simulink model "Simulations_chapter5_method2"  (R2023a)
settings: Solver=ode23s  StartTime=0.0  StopTime=20  RelTol=1e-3  EnableMultiTasking=on
values from neighbouring files (symbols this model uses):
  Akmax = EstMax.a    [Chapter5_method2.m]
  Akmin = Estmin.a    [Chapter5_method2.m]
  Bkmax = EstMax.b    [Chapter5_method2.m]
  Bkmin = Estmin.b    [Chapter5_method2.m]
  c0 = 68.83    [Chapter5_method2.m]
  c1 = 21    [Chapter5_method2.m]
  Ckmax = EstMax.c    [Chapter5_method2.m]
  Ckmin = Estmin.c    [Chapter5_method2.m]
  Dkmax = EstMax.d    [Chapter5_method2.m]
  Dkmin = Estmin.d    [Chapter5_method2.m]
  fc = 28.07    [Chapter5_method2.m]
  Fer0 = 1    [Init_simulations_chapter5_method2.m]
  k0 = 170.4    [Chapter5_method2.m]
  k1 = 218.16    [Chapter5_method2.m]
  ks = 1396    [Chapter5_method2.m]
  kt = 12270    [Chapter5_method2.m]
  ms = 2.27    [Chapter5_method2.m]
  mus = 0.25    [Chapter5_method2.m]
  rhomax = 1    [Chapter5_method2.m]
  rhomin = -1    [Chapter5_method2.m]
  scenario = input('Which scenario would you like to run: 1, 2 or 3? Answer = ')    [Init_simulations_chapter5_method2.m]
  tau = 43e-3    (= 0.043)    [Chapter5_method2.m]
  Ts = 0.005    [Init_simulations_chapter5_method2.m]
  umax = 0.35    [Init_simulations_chapter5_method2.m]
  umin = 0.1    [Init_simulations_chapter5_method2.m]
  zs0 = 0.001    [Init_simulations_chapter5_method2.m]
  zsdt0 = 0.001    [Init_simulations_chapter5_method2.m]
  zus0 = 0.001    [Init_simulations_chapter5_method2.m]
  zusdt0 = 0.001    [Init_simulations_chapter5_method2.m]
libraries: simulink x4
settings Model: Creator=aestr  LastModifiedBy=senameo
settings SolverCC: AlgebraicLoopSolver=TrustRegion
settings DataIOCC: LimitDataPoints=on  SaveFormat=Array  ReturnWorkspaceOutputs=off
settings OptimizationCC: LifeSpan=inf
settings DebuggingCC: UnconnectedInputMsg=warning  UnconnectedOutputMsg=warning  UnconnectedLineMsg=warning  SFUnexpectedBacktrackingDiag=warning  SFNoUnconditionalDefaultTransitionDiag=warning  SFExecutionAtInitializationDiag=none  ArithmeticOperatorsInVariantConditions=warning
settings HardwareCC: ProdBitPerPointer=32  ProdBitPerSizeT=32  ProdBitPerPtrDiffT=32  ProdLargestAtomicFloat=None  ProdIntDivRoundTo=Undefined  ProdEndianess=Unspecified  ProdWordSize=32  ProdHWDeviceType=32-bit Generic
settings ModelReferenceCC: EnableRefExpFcnMdlSchedulingChecks=on  PropagateSignalLabelsOutOfModel=off
settings SFSimCC: SimUseLocalCustomCode=off  CustomCodeUndefinedFunction=UseInterfaceOnly
settings RTWCC: RTWUseLocalCustomCode=off  DLArmComputeVersion=19.05
settings CodeAppCC: StateflowObjectComments=on
settings GRTTargetCC: TargetLangStandard=C89/C90 (ANSI)
settings ConfigComp: CovMetricSettings=dw  CovSaveCumulativeToWorkspaceVar=on  CovSaveSingleToWorkspaceVar=on  CovExternalEMLEnable=off

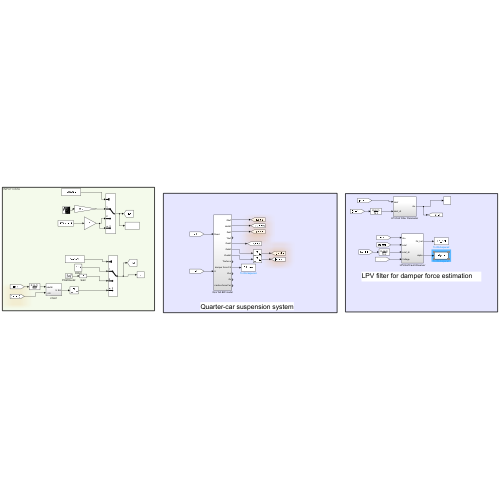
[thumbnail: Simulink's stored preview of the top-level diagram]
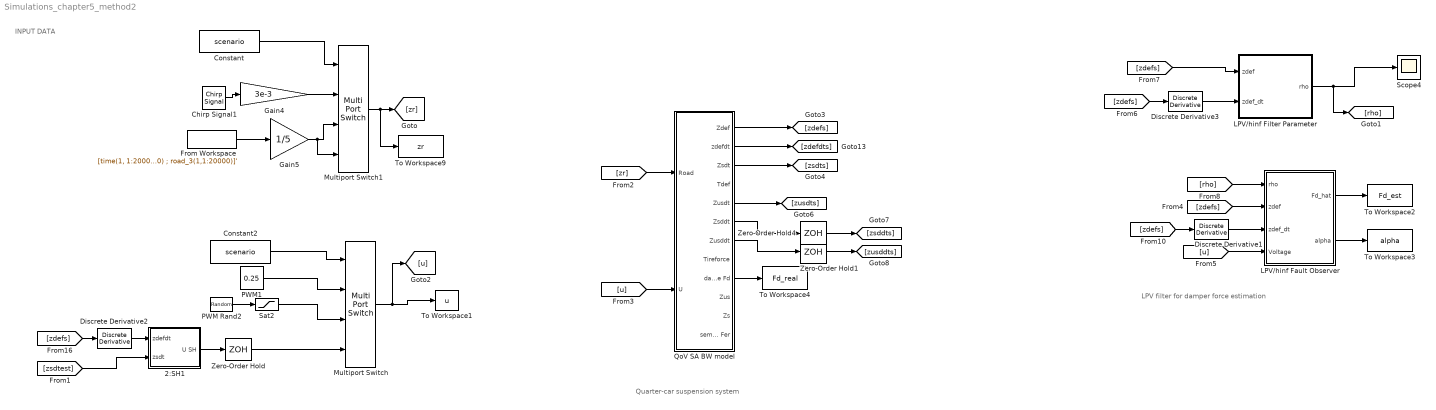
== system Simulations_chapter5_method2 ==
  note: INPUT DATA
  note: Quarter-car suspension system
  note: LPV filter for damper force estimation
  2:SH1 : Subsystem  AncestorBlock=controladores/Hybrid Controller/Sky Hook
  Chirp Signal1 : simulink/Sources/Chirp Signal  f1=0  T=20  f2=10
  Constant : Constant  Value=scenario
  Constant2 : Constant  Value=scenario
  Discrete Derivative1 : simulink/Discrete/Discrete Derivative  gainval=1.0  ICPrevScaledInput=0.0  OutMin=[]  OutMax=[]  OutDataType=fixdt(1, 16)  OutScaling=2^-10  DoSatur=off
  Discrete Derivative2 : simulink/Discrete/Discrete Derivative  gainval=1.0  ICPrevScaledInput=0.0  OutMin=[]  OutMax=[]  OutDataType=fixdt(1, 16)  OutScaling=2^-10  DoSatur=off
  Discrete Derivative3 : simulink/Discrete/Discrete Derivative  gainval=1.0  ICPrevScaledInput=0.0  OutMin=[]  OutMax=[]  OutDataType=fixdt(1, 16)  OutScaling=2^-10  DoSatur=off
  From Workspace : FromWorkspace  VariableName=[time(1, 1:20000) ; road_3(1,1:20000)]'
  Gain4 : Gain  Gain=3e-3
  Gain5 : Gain  Gain=1/5
  LPV/hinf Fault Observer : Subsystem
  LPV/hinf Filter Parameter : Subsystem
  Multiport Switch : MultiPortSwitch  SaturateOnIntegerOverflow=off  InputSameDT=off
  Multiport Switch1 : MultiPortSwitch  SaturateOnIntegerOverflow=off  InputSameDT=off
  PWM Rand2 : UniformRandomNumber  Minimum=0.05  Maximum=0.4  Seed=5  SampleTime=2
  PWM1 : Constant  Value=0.25
  QoV SA BW model : Subsystem
  Sat2 : Saturate  UpperLimit=0.35  LowerLimit=0.1
  Scope4 : Scope
  To Workspace1 : ToWorkspace  VariableName=u  SaveFormat=Structure With Time  SampleTime=-1
  To Workspace2 : ToWorkspace  VariableName=Fd_est  SaveFormat=Structure With Time  SampleTime=-1
  To Workspace3 : ToWorkspace  VariableName=alpha  SaveFormat=Structure With Time  SampleTime=-1
  To Workspace4 : ToWorkspace  VariableName=Fd_real  SaveFormat=Structure With Time  SampleTime=-1
  To Workspace9 : ToWorkspace  VariableName=zr  SaveFormat=Structure With Time  SampleTime=-1
  Zero-Order Hold : ZeroOrderHold  SampleTime=Ts
  Zero-Order Hold1 : ZeroOrderHold  SampleTime=Ts
  Zero-Order Hold4 : ZeroOrderHold  SampleTime=Ts
  wires:
  QoV SA BW model/3(Zsdt) -> [zsdts]
  QoV SA BW model/5(Zusdt) -> [zusdts]
  QoV SA BW model/7(Zusddt) -> Zero-Order Hold1/1
  Zero-Order Hold4/1 -> [zsddts]
  Zero-Order Hold1/1 -> [zusddts]
  QoV SA BW model/9(damper force Fd) -> To Workspace4/1
  QoV SA BW model/2(zdefdt) -> [zdefdts]
  QoV SA BW model/1(Zdef) -> [zdefs]
  QoV SA BW model/6(Zsddt) -> Zero-Order Hold4/1
  Multiport Switch1/1 -> To Workspace9/1, [zr]
  Chirp Signal1/1 -> Gain4/1
  [zr] -> QoV SA BW model/1(Road)
  [u] -> QoV SA BW model/2(U)
  [zdefs] -> Discrete Derivative2/1
  Discrete Derivative2/1 -> 2:SH1/1(zdefdt)
  [zsdtest] -> 2:SH1/2(zsdt)
  Constant2/1 -> Multiport Switch/1
  2:SH1/1(U SH) -> Zero-Order Hold/1
  Sat2/1 -> Multiport Switch/3
  PWM1/1 -> Multiport Switch/2
  Multiport Switch/1 -> To Workspace1/1, [u]
  Zero-Order Hold/1 -> Multiport Switch/4
  PWM Rand2/1 -> Sat2/1
  Constant/1 -> Multiport Switch1/1
  Gain4/1 -> Multiport Switch1/2
  From Workspace/1 -> Gain5/1
  Gain5/1 -> Multiport Switch1/4, Multiport Switch1/3
  Discrete Derivative3/1 -> LPV/hinf Filter Parameter/2(zdef_dt)
  [zdefs] -> Discrete Derivative3/1
  LPV/hinf Filter Parameter/1(rho) -> [rho], Scope4/1
  [zdefs] -> LPV/hinf Filter Parameter/1(zdef)
  Discrete Derivative1/1 -> LPV/hinf Fault Observer/3(zdef_dt)
  [zdefs] -> LPV/hinf Fault Observer/2(zdef)
  [zdefs] -> Discrete Derivative1/1
  [u] -> LPV/hinf Fault Observer/4(Voltage)
  [rho] -> LPV/hinf Fault Observer/1(rho)
  LPV/hinf Fault Observer/1(Fd_hat) -> To Workspace2/1
  LPV/hinf Fault Observer/2(alpha) -> To Workspace3/1

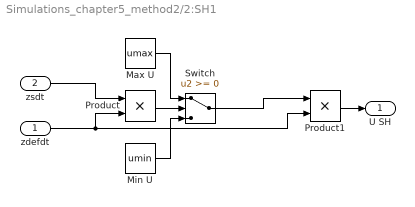
== system Simulations_chapter5_method2/2:SH1 ==
  zdefdt : Inport
  zsdt : Inport  Port=2
  Max U : Constant  Value=umax
  Min U : Constant  Value=umin
  Product : Product  RndMeth=Zero
  Product1 : Product  RndMeth=Zero
  Switch : Switch  SaturateOnIntegerOverflow=off  InputSameDT=off
  U SH : Outport  VectorParamsAs1DForOutWhenUnconnected=off
  wires:
  zsdt/1 -> Product/1
  zdefdt/1 -> Product1/2, Product/2
  Max U/1 -> Switch/1
  Min U/1 -> Switch/3
  Product/1 -> Switch/2
  Switch/1 -> Product1/1
  Product1/1 -> U SH/1

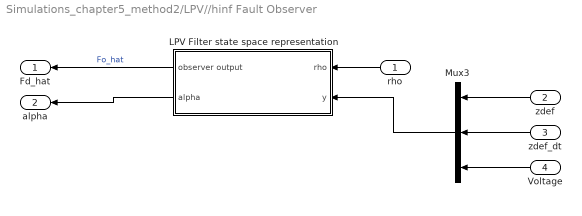
== system Simulations_chapter5_method2/LPV//hinf Fault Observer ==
  rho : Inport
  zdef : Inport  Port=2
  zdef_dt : Inport  Port=3
  Voltage : Inport  Port=4
  LPV Filter state space representation : Subsystem
  Mux3 : Mux  Inputs=3
  Fd_hat : Outport
  alpha : Outport  Port=2
  wires:
  Mux3/1 -> LPV Filter state space representation/2(y)
  LPV Filter state space representation/1(observer output) -> Fd_hat/1  "Fo_hat"
  Voltage/1 -> Mux3/3
  zdef/1 -> Mux3/1
  zdef_dt/1 -> Mux3/2
  LPV Filter state space representation/2(alpha) -> alpha/1
  rho/1 -> LPV Filter state space representation/1(rho)

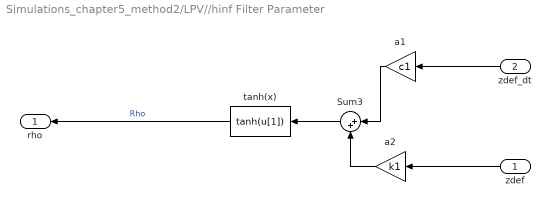
== system Simulations_chapter5_method2/LPV//hinf Filter Parameter ==
  zdef : Inport
  zdef_dt : Inport  Port=2
  Sum3 : Sum  Inputs=|++
  a1 : Gain  Gain=c1
  a2 : Gain  Gain=k1
  tanh(x) : Fcn  Expr=tanh(u[1])
  rho : Outport
  wires:
  Sum3/1 -> tanh(x)/1
  a2/1 -> Sum3/2
  a1/1 -> Sum3/1
  tanh(x)/1 -> rho/1  "Rho"
  zdef/1 -> a2/1
  zdef_dt/1 -> a1/1

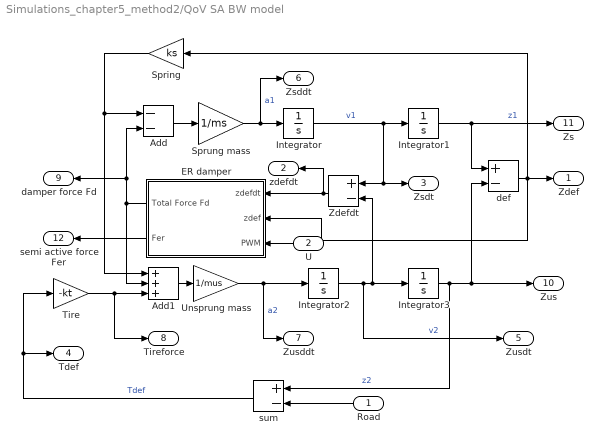
== system Simulations_chapter5_method2/QoV SA BW model ==
  Road : Inport
  U : Inport  Port=2
  Add : Sum  Inputs=--
  Add1 : Sum  Inputs=+++
  ER damper : Subsystem
  Integrator : Integrator  InitialCondition=zsdt0
  Integrator1 : Integrator  InitialCondition=zs0
  Integrator2 : Integrator  InitialCondition=zusdt0
  Integrator3 : Integrator  InitialCondition=zus0
  Spring : Gain  Gain=ks
  Sprung mass : Gain  Gain=1/ms
  Tire : Gain  Gain=-kt
  Unsprung mass : Gain  Gain=1/mus
  Zdefdt : Sum  Inputs=+-
  def : Sum  Inputs=+-
  sum : Sum  Inputs=+-
  Zdef : Outport
  zdefdt : Outport  Port=2
  Zsdt : Outport  Port=3
  Tdef : Outport  Port=4
  Zusdt : Outport  Port=5
  Zsddt : Outport  Port=6
  Zusddt : Outport  Port=7
  Tireforce : Outport  Port=8
  damper force Fd : Outport  Port=9
  Zus : Outport  Port=10
  Zs : Outport  Port=11
  semi active force Fer : Outport  Port=12
  wires:
  Integrator/1 -> Zsdt/1, Zdefdt/1, Integrator1/1  "v1"
  Integrator2/1 -> Zusdt/1, Zdefdt/2, Integrator3/1  "v2"
  Sprung mass/1 -> Zsddt/1, Integrator/1  "a1"
  Unsprung mass/1 -> Zusddt/1, Integrator2/1  "a2"
  Add/1 -> Sprung mass/1
  Add1/1 -> Unsprung mass/1
  Integrator1/1 -> def/1, Zs/1  "z1"
  Integrator3/1 -> sum/1, def/2, Zus/1  "z2"
  def/1 -> ER damper/2(zdef), Zdef/1, Spring/1
  Spring/1 -> Add/1, Add1/1
  Tire/1 -> Tireforce/1, Add1/3
  Road/1 -> sum/2
  sum/1 -> Tdef/1, Tire/1  "Tdef"
  ER damper/1(Total Force Fd) -> Add1/2, Add/2, damper force Fd/1
  U/1 -> ER damper/3(PWM)
  Zdefdt/1 -> ER damper/1(zdefdt), zdefdt/1
  ER damper/2(Fer) -> semi active force Fer/1

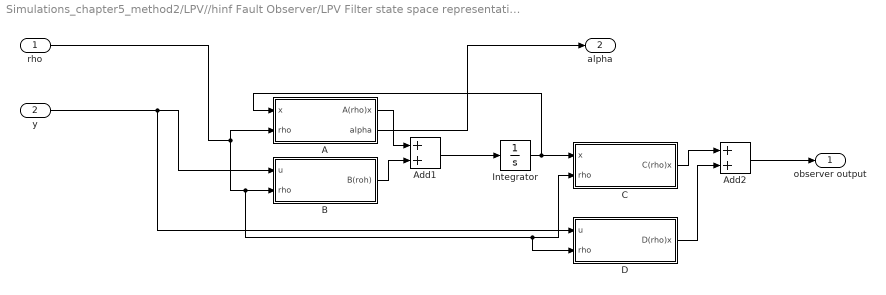
== system Simulations_chapter5_method2/LPV//hinf Fault Observer/LPV Filter state space representation ==
  rho : Inport
  y : Inport  Port=2
  A : Subsystem
  Add1 : Sum
  Add2 : Sum
  B : Subsystem
  C : Subsystem
  D : Subsystem
  Integrator : Integrator
  observer output : Outport  VectorParamsAs1DForOutWhenUnconnected=off
  alpha : Outport  Port=2  VectorParamsAs1DForOutWhenUnconnected=off
  wires:
  A/2(alpha) -> alpha/1
  C/1(C(rho)x) -> Add2/1
  D/1(D(rho)x) -> Add2/2
  Integrator/1 -> C/1(x), A/1(x)
  Add1/1 -> Integrator/1
  B/1(B(roh)) -> Add1/2
  A/1(A(rho)x) -> Add1/1
  rho/1 -> A/2(rho), B/2(rho), C/2(rho), D/2(rho)
  Add2/1 -> observer output/1
  y/1 -> B/1(u), D/1(u)

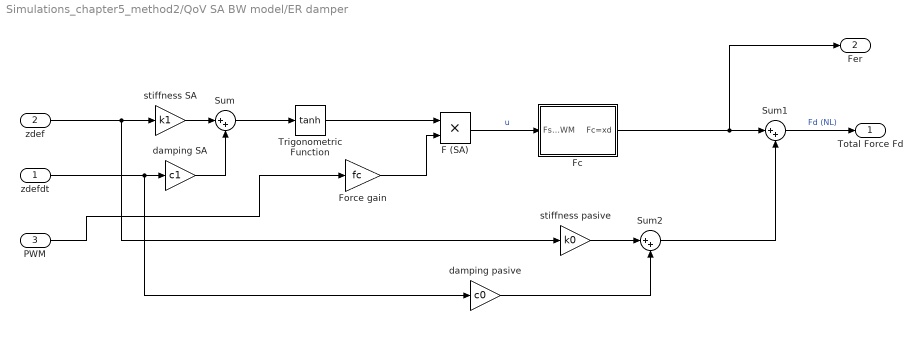
== system Simulations_chapter5_method2/QoV SA BW model/ER damper ==
  zdefdt : Inport
  zdef : Inport  Port=2
  PWM : Inport  Port=3
  "F (SA) " : Product  RndMeth=Zero
  Fc : Subsystem
  Force gain : Gain  Gain=fc
  Sum : Sum  Inputs=|++
  Sum1 : Sum  Inputs=|++
  Sum2 : Sum  Inputs=|++
  Trigonometric Function : Trigonometry  Operator=tanh
  damping SA : Gain  Gain=c1
  damping pasive : Gain  Gain=c0
  stiffness SA : Gain  Gain=k1
  stiffness pasive : Gain  Gain=k0
  Total Force Fd : Outport
  Fer : Outport  Port=2
  wires:
  zdefdt/1 -> damping pasive/1, damping SA/1
  stiffness SA/1 -> Sum/1
  damping SA/1 -> Sum/2
  Sum/1 -> Trigonometric Function/1
  Trigonometric Function/1 -> "F (SA) "/1
  PWM/1 -> Force gain/1
  Force gain/1 -> "F (SA) "/2
  stiffness pasive/1 -> Sum2/1
  damping pasive/1 -> Sum2/2
  "F (SA) "/1 -> Fc/1(Fsa*PWM)  "u"
  Fc/1(Fc=xd) -> Fer/1, Sum1/1
  Sum2/1 -> Sum1/2
  Sum1/1 -> Total Force Fd/1  "Fd (NL)"
  zdef/1 -> stiffness pasive/1, stiffness SA/1

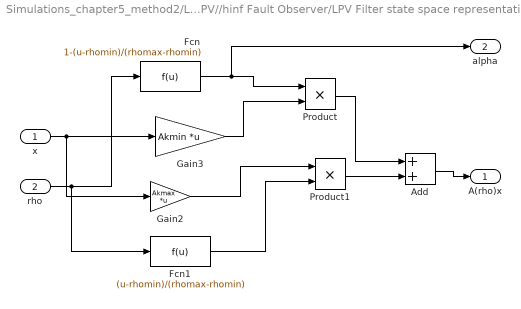
== system Simulations_chapter5_method2/LPV//hinf Fault Observer/LPV Filter state space representation/A ==
  x : Inport
  rho : Inport  Port=2
  Add : Sum
  Fcn : Fcn  Expr=1-(u-rhomin)/(rhomax-rhomin)
  Fcn1 : Fcn  Expr=(u-rhomin)/(rhomax-rhomin)
  Gain2 : Gain  Gain=Akmax  Multiplication=Matrix(K*u)
  Gain3 : Gain  Gain=Akmin  Multiplication=Matrix(K*u)
  Product : Product
  Product1 : Product
  A(rho)x : Outport  VectorParamsAs1DForOutWhenUnconnected=off
  alpha : Outport  Port=2  VectorParamsAs1DForOutWhenUnconnected=off
  wires:
  x/1 -> Gain3/1, Gain2/1
  rho/1 -> Fcn/1, Fcn1/1
  Product/1 -> Add/1
  Product1/1 -> Add/2
  Add/1 -> A(rho)x/1
  Fcn/1 -> Product/1, alpha/1
  Fcn1/1 -> Product1/2
  Gain3/1 -> Product/2
  Gain2/1 -> Product1/1

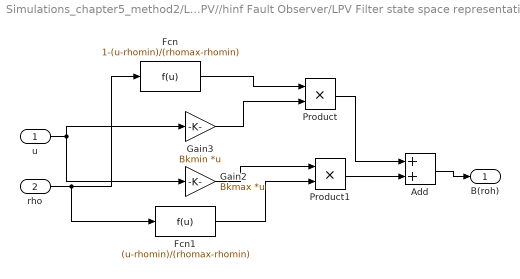
== system Simulations_chapter5_method2/LPV//hinf Fault Observer/LPV Filter state space representation/B ==
  u : Inport
  rho : Inport  Port=2
  Add : Sum
  Fcn : Fcn  Expr=1-(u-rhomin)/(rhomax-rhomin)
  Fcn1 : Fcn  Expr=(u-rhomin)/(rhomax-rhomin)
  Gain2 : Gain  Gain=Bkmax  Multiplication=Matrix(K*u)
  Gain3 : Gain  Gain=Bkmin  Multiplication=Matrix(K*u)
  Product : Product
  Product1 : Product
  B(roh) : Outport  VectorParamsAs1DForOutWhenUnconnected=off
  wires:
  u/1 -> Gain3/1, Gain2/1
  rho/1 -> Fcn/1, Fcn1/1
  Product/1 -> Add/1
  Product1/1 -> Add/2
  Add/1 -> B(roh)/1
  Fcn/1 -> Product/1
  Fcn1/1 -> Product1/2
  Gain3/1 -> Product/2
  Gain2/1 -> Product1/1

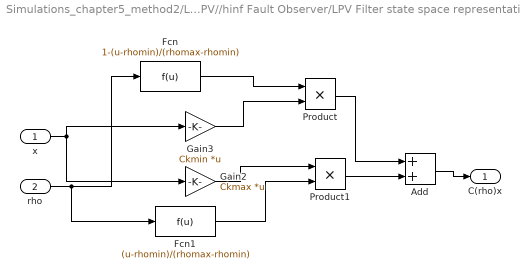
== system Simulations_chapter5_method2/LPV//hinf Fault Observer/LPV Filter state space representation/C ==
  x : Inport
  rho : Inport  Port=2
  Add : Sum
  Fcn : Fcn  Expr=1-(u-rhomin)/(rhomax-rhomin)
  Fcn1 : Fcn  Expr=(u-rhomin)/(rhomax-rhomin)
  Gain2 : Gain  Gain=Ckmax  Multiplication=Matrix(K*u)
  Gain3 : Gain  Gain=Ckmin  Multiplication=Matrix(K*u)
  Product : Product
  Product1 : Product
  C(rho)x : Outport  VectorParamsAs1DForOutWhenUnconnected=off
  wires:
  x/1 -> Gain3/1, Gain2/1
  rho/1 -> Fcn/1, Fcn1/1
  Product/1 -> Add/1
  Product1/1 -> Add/2
  Add/1 -> C(rho)x/1
  Fcn/1 -> Product/1
  Fcn1/1 -> Product1/2
  Gain3/1 -> Product/2
  Gain2/1 -> Product1/1

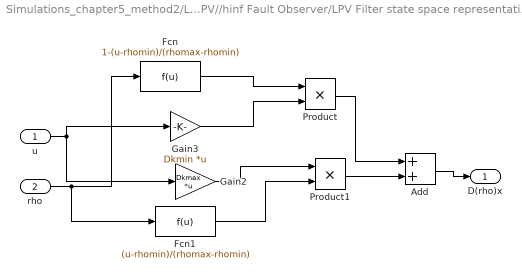
== system Simulations_chapter5_method2/LPV//hinf Fault Observer/LPV Filter state space representation/D ==
  u : Inport
  rho : Inport  Port=2
  Add : Sum
  Fcn : Fcn  Expr=1-(u-rhomin)/(rhomax-rhomin)
  Fcn1 : Fcn  Expr=(u-rhomin)/(rhomax-rhomin)
  Gain2 : Gain  Gain=Dkmax  Multiplication=Matrix(K*u)
  Gain3 : Gain  Gain=Dkmin  Multiplication=Matrix(K*u)
  Product : Product
  Product1 : Product
  D(rho)x : Outport  VectorParamsAs1DForOutWhenUnconnected=off
  wires:
  u/1 -> Gain3/1, Gain2/1
  rho/1 -> Fcn/1, Fcn1/1
  Product/1 -> Add/1
  Product1/1 -> Add/2
  Add/1 -> D(rho)x/1
  Fcn/1 -> Product/1
  Fcn1/1 -> Product1/2
  Gain3/1 -> Product/2
  Gain2/1 -> Product1/1

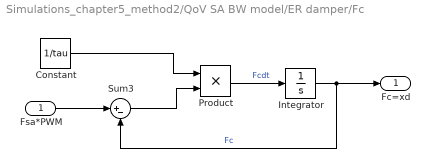
== system Simulations_chapter5_method2/QoV SA BW model/ER damper/Fc ==
  Fsa*PWM : Inport
  Constant : Constant  Value=1/tau
  Integrator : Integrator  InitialCondition=Fer0
  Product : Product  RndMeth=Zero
  Sum3 : Sum  Inputs=|+-
  Fc=xd : Outport
  wires:
  Integrator/1 -> Sum3/2, Fc=xd/1  "Fc"
  Fsa*PWM/1 -> Sum3/1
  Sum3/1 -> Product/2
  Product/1 -> Integrator/1  "Fcdt"
  Constant/1 -> Product/1
